simulink model "DinamicaTesis"  (R2021b)
settings: Solver=VariableStepAuto  StartTime=0.0  StopTime=50  RelTol=1e-3
(part 1 of 3)
settings Model: Creator=fabia  LastModifiedBy=fabia

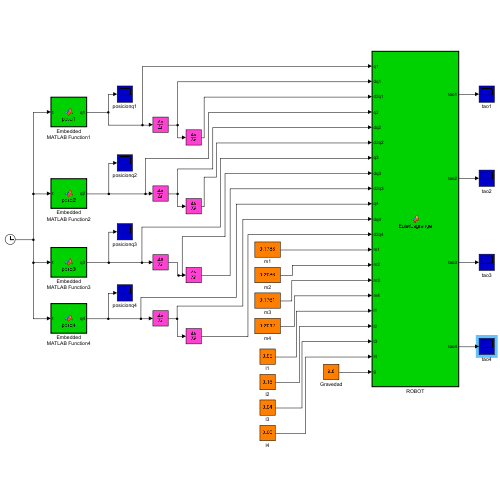
[thumbnail: Simulink's stored preview of the top-level diagram]
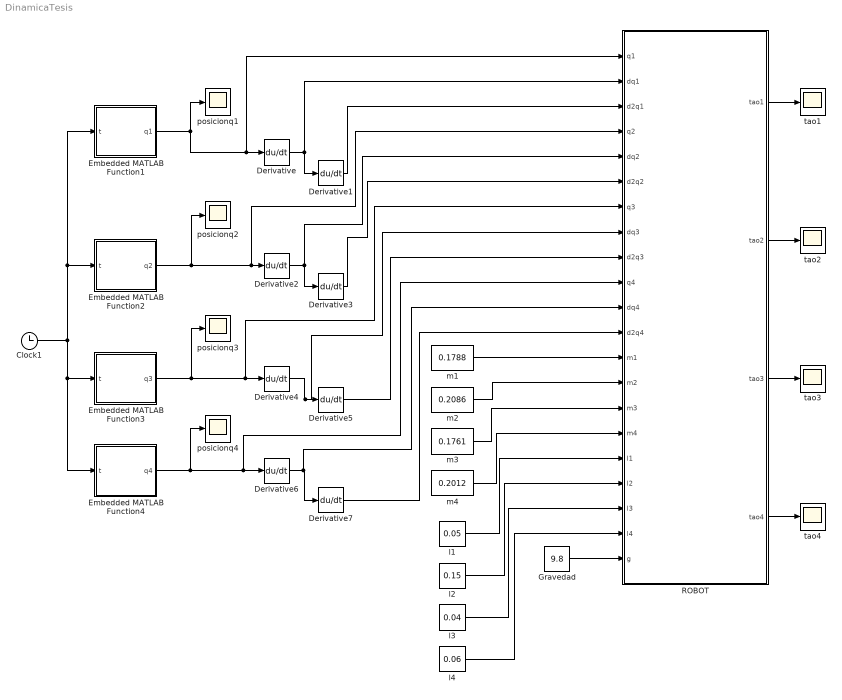
== system DinamicaTesis ==
  Clock1 : Clock
      settings: Decimation=1000
  Derivative{,1..7} (8 alike) : Derivative
  Embedded MATLAB Function1 : MATLAB Function  TreatAsAtomicUnit=on
  Embedded MATLAB Function2 : MATLAB Function  TreatAsAtomicUnit=on
  Embedded MATLAB Function3 : MATLAB Function  TreatAsAtomicUnit=on
  Embedded MATLAB Function4 : MATLAB Function  TreatAsAtomicUnit=on
  Gravedad : Constant  Value=9.8
  ROBOT : MATLAB Function  TreatAsAtomicUnit=on
  l1 : Constant  Value=0.05
  l2 : Constant  Value=0.15
  l3 : Constant  Value=0.04
  l4 : Constant  Value=0.06
  m1 : Constant  Value=0.1788
  m2 : Constant  Value=0.2086
  m3 : Constant  Value=0.1761
  m4 : Constant  Value=0.2012
  posicionq{1..4} (4 alike) : Scope
  tao{1..4} (4 alike) : Scope
  wires:
  Embedded MATLAB Function3/1(q3) -> posicionq3/1, ROBOT/7(q3), Derivative4/1
  Derivative5/1 -> ROBOT/9(d2q3)
  Derivative/1 -> ROBOT/2(dq1), Derivative1/1
  Derivative4/1 -> ROBOT/8(dq3), Derivative5/1
  Derivative3/1 -> ROBOT/6(d2q2)
  Derivative2/1 -> ROBOT/5(dq2), Derivative3/1
  Derivative1/1 -> ROBOT/3(d2q1)
  Embedded MATLAB Function2/1(q2) -> posicionq2/1, ROBOT/4(q2), Derivative2/1
  Embedded MATLAB Function1/1(q1) -> ROBOT/1(q1), Derivative/1, posicionq1/1
  ROBOT/2(tao2) -> tao2/1
  ROBOT/1(tao1) -> tao1/1
  ROBOT/3(tao3) -> tao3/1
  Gravedad/1 -> ROBOT/21(g)
  m1/1 -> ROBOT/13(m1)
  m2/1 -> ROBOT/14(m2)
  m3/1 -> ROBOT/15(m3)
  l1/1 -> ROBOT/17(l1)
  l2/1 -> ROBOT/18(l2)
  l3/1 -> ROBOT/19(l3)
  Clock1/1 -> Embedded MATLAB Function2/1(t), Embedded MATLAB Function1/1(t), Embedded MATLAB Function4/1(t), Embedded MATLAB Function3/1(t)
  l4/1 -> ROBOT/20(l4)
  Embedded MATLAB Function4/1(q4) -> posicionq4/1, ROBOT/10(q4), Derivative6/1
  Derivative6/1 -> ROBOT/11(dq4), Derivative7/1
  Derivative7/1 -> ROBOT/12(d2q4)
  ROBOT/4(tao4) -> tao4/1
  m4/1 -> ROBOT/16(m4)

== matlab function DinamicaTesis/Embedded MATLAB Function4 ==
  data: q4 output; t input
function q4 = posq4(t)
% This block supports an embeddable subset of the MATLAB language.
% See the help menu for details. 

if (t>=17)  % Si el t>=tmax, se repite una vez la rutina
    t=t-17;
end

if(t<6) % Movimiento 1
    t_inic = 0; % Tiempo en que inicia
    tf = 4;     % Tiempo en que termina
    y_ini = 1.570;
    y_f = -0.785;
elseif (t>=6 && t<12) % Movimiento 2
    t_inic = 6;
    tf = 4;
    y_ini = -0.785;
    y_f = -0.785;
else  % Movimiento 3
    t_inic = 12;
    tf = 5;
    y_ini = -0.785;
    y_f =  1.570;
end

% Calculo de trayectoria de tiempo minimo
Tb = tf/2;
% Vmax = 2*(y_f - y_ini)/(tf);
Vmax = (y_f - y_ini)/(tf - Tb);
ta = t - t_inic;
if(ta<0)
    q4 = y_ini;
elseif(ta >= 0 && ta < Tb)
    q4 = y_ini + (Vmax/(2*Tb))*ta*ta;
elseif(ta >= Tb && ta < (tf - Tb))
    q4 = (y_ini + y_f - Vmax*tf)/2 + Vmax*ta;
elseif(ta >= (tf - Tb) && ta < tf)
     q4 = y_f - (Vmax*(tf-ta)*(tf-ta)/(2*Tb));
else
    q4 = y_f;
end

== matlab function DinamicaTesis/Embedded MATLAB Function1 ==
  data: q1 output; t input
function q1 = posq1(t)
% This block supports an embeddable subset of the MATLAB language.
% See the help menu for details. 

if (t>=17)  % Si el t>=tmax, se repite otra vez la rutina
    t=t-17;
end

if(t<6) % Movimiento 1
    t_inic = 0; % Tiempo en que inicia
    tf = 4;     % Tiempo en que termina
    y_ini = 0;  % Posicion articular inicial (rad)
    y_f = -3.14159;    % Posicion articular final (rad)
elseif (t>=6 && t<12) % Movimiento 2
    t_inic = 6;
    tf = 4;
    y_ini = -3.14159;
    y_f =-3.14159;
else  % Movimiento 3
    t_inic = 12;
    tf = 5;
    y_ini =-3.14159;
    y_f = 0;
end

% Calculo de trayectoria de tiempo minimo
Tb = tf/2;  % el tb queda a la mitad del tiempo final

% Vmax = 2*(y_f - y_ini)/(tf);

Vmax = (y_f - y_ini)/(tf - Tb);
ta = t - t_inic;

% Polinomios que describen la curva en funcion de tiempo
if(ta<0)
    q1 = y_ini;
elseif(ta >= 0 && ta < Tb)
    q1 = y_ini + (Vmax/(2*Tb))*ta*ta;
elseif(ta >= Tb && ta < (tf - Tb))
    q1 = (y_ini + y_f - Vmax*tf)/2 + Vmax*ta;
elseif(ta >= (tf - Tb) && ta < tf)
     q1 = y_f - (Vmax*(tf-ta)*(tf-ta)/(2*Tb));
else
    q1 = y_f;
end

== matlab function DinamicaTesis/Embedded MATLAB Function2 ==
  data: q2 output; t input
function q2 = posq2(t)
% This block supports an embeddable subset of the MATLAB language.
% See the help menu for details. 

if (t>=17)  % Si el t>=tmax, se repite una vez la rutina
    t=t-17;
end

if(t<6) % Movimiento 1
    t_inic = 0; % Tiempo en que inicia
    tf = 4;     % Tiempo en que termina
    y_ini = 0.785;
    y_f = -1.570;
elseif (t>=6 && t<12) % Movimiento 2
    t_inic = 6;
    tf = 4;
    y_ini =  -1.5706;
    y_f =  -1.570;
else  % Movimiento 3
    t_inic = 12;
    tf = 5;
    y_ini =  -1.570;
    y_f = 0.785;
end

% Calculo de trayectoria de tiempo minimo
Tb = tf/2;
% Vmax = 2*(y_f - y_ini)/(tf);
Vmax = (y_f - y_ini)/(tf - Tb);
ta = t - t_inic;
if(ta<0)
    q2 = y_ini;
elseif(ta >= 0 && ta < Tb)
    q2 = y_ini + (Vmax/(2*Tb))*ta*ta;
elseif(ta >= Tb && ta < (tf - Tb))
    q2 = (y_ini + y_f - Vmax*tf)/2 + Vmax*ta;
elseif(ta >= (tf - Tb) && ta < tf)
     q2 = y_f - (Vmax*(tf-ta)*(tf-ta)/(2*Tb));
else
    q2 = y_f;
end
